simulink library "ammclib_bam"  (Simulink 9.3)
settings: Solver=VariableStepAuto  StartTime=0.0  StopTime=10.0  RelTol=1e-3
undefined symbols (not defined in the file or in its folder): f16A1, f16A2, f16ADCMaxError, f16B0, f16B1, f16B2, f16C1, f16CC1, f16CC1sc, f16CC1sc_D, f16CC1sc_Q, f16CC2, f16CC2sc, f16CC2sc_D, f16CC2sc_Q, f16DerivGain, f16EGain, f16FiltCoef, f16HystOff, f16HystOn, f16IGain, f16IntegGain, f16IntegGainFW, f16IntegGainQ, f16Kd, f16Kq, f16Limit, f16LowerLimit, f16LowerLimit_D, f16LowerLimit_Q, f16LowerLimitFW, f16LowerLimitQ, f16ModIndex, f16OutValOff, f16OutValOn, f16PropGain, f16PropGainFW, f16PropGainQ, f16RampDown, f16RampUp, f16UGain, f16UpperLimit, f16UpperLimit_D, f16UpperLimit_Q, f16UpperLimitFW, f16UpperLimitQ, f16WIGain, f32A1, f32A2, f32ADCMaxError, f32B0, f32B1, f32B2, f32C1, f32CC1, f32CC1sc, f32CC1sc_D, f32CC1sc_Q, f32CC2, f32CC2sc ... (+114)
(part 18 of 21)

== system ammclib_bam/GFLIB/F32/GFLIB_Asin_F32 ==
  f32In : Inport  OutDataTypeStr=int32
  GFLIB_Asin_SF : S-Function  FunctionName=GFLIB_Asin_SF_F32  SFunctionDeploymentMode=off  EnableBusSupport=off
  copyright : Subsystem
      mask Display: text(10,90,'FILE:');text(10,75,'DESRIPTION:');text(10,60,'COPYRIGHT:');text(10,45,'VERSION:');text(10,30,'DATE:')
  copyright2 : Subsystem
      mask Display: text(10,90,'GFLIB_Asin_BAM_F32.mdl');text(10,75,'Inverse sine function');text(10,60,'NXP 2020');text(10,45,'1.0');text(10,30,'18-Mar-2020');
  f32Out : Outport
  wires:
  GFLIB_Asin_SF/1 -> f32Out/1
  f32In/1 -> GFLIB_Asin_SF/1

== system ammclib_bam/GFLIB/F32/GFLIB_AtanYXShifted_F32 ==
  f32InY : Inport  OutDataTypeStr=int32
  f32InX : Inport  Port=2  OutDataTypeStr=int32
  Ky : Inport  Port=3  OutDataTypeStr=int32
  Kx : Inport  Port=4  OutDataTypeStr=int32
  Ny : Inport  Port=5  OutDataTypeStr=int32
  Nx : Inport  Port=6  OutDataTypeStr=int32
  ThetaAdj : Inport  Port=7  OutDataTypeStr=int32
  GFLIB_AtanYXShifted_SF : S-Function  FunctionName=GFLIB_AtanYXShifted_SF_F32  SFunctionDeploymentMode=off  EnableBusSupport=off
  copyright : Subsystem
      mask Display: text(10,90,'FILE:');text(10,75,'DESRIPTION:');text(10,60,'COPYRIGHT:');text(10,45,'VERSION:');text(10,30,'DATE:')
  copyright2 : Subsystem
      mask Display: text(10,90,'GFLIB_AtanYXShifted_BAM_F32.mdl');text(10,75,'Shifted arctangent of two arguments Y/X.');text(10,60,'NXP 2020');text(10,45,'1.0');text(10,30,'18-Mar-2020');
  f32Out : Outport
  wires:
  GFLIB_AtanYXShifted_SF/1 -> f32Out/1
  ThetaAdj/1 -> GFLIB_AtanYXShifted_SF/7
  Nx/1 -> GFLIB_AtanYXShifted_SF/6
  Ny/1 -> GFLIB_AtanYXShifted_SF/5
  Kx/1 -> GFLIB_AtanYXShifted_SF/4
  Ky/1 -> GFLIB_AtanYXShifted_SF/3
  f32InX/1 -> GFLIB_AtanYXShifted_SF/2
  f32InY/1 -> GFLIB_AtanYXShifted_SF/1

== system ammclib_bam/GFLIB/F32/GFLIB_AtanYX_F32 ==
  f32InY : Inport  OutDataTypeStr=int32
  f32InX : Inport  Port=2  OutDataTypeStr=int32
  GFLIB_AtanYX_SF : S-Function  FunctionName=GFLIB_AtanYX_SF_F32  SFunctionDeploymentMode=off  EnableBusSupport=off
  copyright : Subsystem
      mask Display: text(10,90,'FILE:');text(10,75,'DESRIPTION:');text(10,60,'COPYRIGHT:');text(10,45,'VERSION:');text(10,30,'DATE:')
  copyright2 : Subsystem
      mask Display: text(10,90,'GFLIB_AtanYX_BAM_F32.mdl');text(10,75,'Arctangent of two arguments Y/X.');text(10,60,'NXP 2020');text(10,45,'1.0');text(10,30,'18-Mar-2020');
  f32Out : Outport
  wires:
  GFLIB_AtanYX_SF/1 -> f32Out/1
  f32InX/1 -> GFLIB_AtanYX_SF/2
  f32InY/1 -> GFLIB_AtanYX_SF/1

== system ammclib_bam/GFLIB/F32/GFLIB_Atan_F32 ==
  f32In : Inport  OutDataTypeStr=int32
  GFLIB_Atan_SF : S-Function  FunctionName=GFLIB_Atan_SF_F32  SFunctionDeploymentMode=off  EnableBusSupport=off
  copyright : Subsystem
      mask Display: text(10,90,'FILE:');text(10,75,'DESRIPTION:');text(10,60,'COPYRIGHT:');text(10,45,'VERSION:');text(10,30,'DATE:')
  copyright2 : Subsystem
      mask Display: text(10,90,'GFLIB_Atan_BAM_F32.mdl');text(10,75,'Inverse tangent function');text(10,60,'NXP 2020');text(10,45,'1.0');text(10,30,'18-Mar-2020');
  f32Out : Outport
  wires:
  GFLIB_Atan_SF/1 -> f32Out/1
  f32In/1 -> GFLIB_Atan_SF/1

== system ammclib_bam/GFLIB/F32/GFLIB_ControllerPIDpAW_F32 ==
  f32InErr : Inport  OutDataTypeStr=int32
  f32ControllerPIDpAWOut_preset : Inport  Port=2  OutDataTypeStr=int32
  Reset : ResetPort  DisableCoverage=on
  GFLIB_ControllerPIDpAW_SF : S-Function  FunctionName=GFLIB_ControllerPIDpAW_SF_F32  Parameters=showStates,resetStatesEnable,f32PropGain,f32IntegGain,f32DerivGain,f32FiltCoef,s16PropGainShift,s16IntegGainShift,s16DerivGainShift,f32LowerLimit,f32UpperLimit  SFunctionDeploymentMode=off  EnableBusSupport=off
  copyright : Subsystem
      mask Display: text(10,90,'FILE:');text(10,75,'DESRIPTION:');text(10,60,'COPYRIGHT:');text(10,45,'VERSION:');text(10,30,'DATE:')
  copyright2 : Subsystem
      mask Display: text(10,90,'GFLIB_ControllerPIDpAW_BAM_F32.mdl');text(10,75,'Parallel form of a standard PID controller with anti-windup.');text(10,60,'NXP 2020');text(10,45,'1.0');text(10,30,'28-Mar-2020');
  f32DerivGain : Ground
  f32DerivPartK_1 : Ground
  f32DerivPartK_1_Out : Terminator
  f32FiltCoef : Ground
  f32InK_1 : Ground
  f32InK_1_Out : Terminator
  f32IntegGain : Ground
  f32IntegPartK_1 : Ground
  f32IntegPartK_1_Out : Terminator
  f32LowerLimit : Ground
  f32PropGain : Ground
  f32UpperLimit : Ground
  s16DerivGainShift : Ground
  s16IntegGainShift : Ground
  s16PropGainShift : Ground
  f32Out : Outport
  u16LimitFlag : Outport  Port=2
  wires:
  GFLIB_ControllerPIDpAW_SF/5 -> f32InK_1_Out/1
  GFLIB_ControllerPIDpAW_SF/4 -> f32DerivPartK_1_Out/1
  GFLIB_ControllerPIDpAW_SF/3 -> f32IntegPartK_1_Out/1
  GFLIB_ControllerPIDpAW_SF/2 -> u16LimitFlag/1
  GFLIB_ControllerPIDpAW_SF/1 -> f32Out/1
  f32InK_1/1 -> GFLIB_ControllerPIDpAW_SF/14
  f32DerivPartK_1/1 -> GFLIB_ControllerPIDpAW_SF/13
  f32IntegPartK_1/1 -> GFLIB_ControllerPIDpAW_SF/12
  f32UpperLimit/1 -> GFLIB_ControllerPIDpAW_SF/11
  f32LowerLimit/1 -> GFLIB_ControllerPIDpAW_SF/10
  s16DerivGainShift/1 -> GFLIB_ControllerPIDpAW_SF/9
  s16IntegGainShift/1 -> GFLIB_ControllerPIDpAW_SF/8
  s16PropGainShift/1 -> GFLIB_ControllerPIDpAW_SF/7
  f32FiltCoef/1 -> GFLIB_ControllerPIDpAW_SF/6
  f32DerivGain/1 -> GFLIB_ControllerPIDpAW_SF/5
  f32IntegGain/1 -> GFLIB_ControllerPIDpAW_SF/4
  f32PropGain/1 -> GFLIB_ControllerPIDpAW_SF/3
  f32ControllerPIDpAWOut_preset/1 -> GFLIB_ControllerPIDpAW_SF/2
  f32InErr/1 -> GFLIB_ControllerPIDpAW_SF/1

== system ammclib_bam/GFLIB/F32/GFLIB_ControllerPIpAW_F32 ==
  f32InErr : Inport  OutDataTypeStr=int32
  f32ControllerPIpAWOut_preset : Inport  Port=2  OutDataTypeStr=int32
  Reset : ResetPort  DisableCoverage=on
  GFLIB_ControllerPIpAW_SF : S-Function  FunctionName=GFLIB_ControllerPIpAW_SF_F32  Parameters=showStates,resetStatesEnable,f32PropGain,f32IntegGain,s16PropGainShift,s16IntegGainShift,f32LowerLimit,f32UpperLimit  SFunctionDeploymentMode=off  EnableBusSupport=off
  copyright : Subsystem
      mask Display: text(10,90,'FILE:');text(10,75,'DESRIPTION:');text(10,60,'COPYRIGHT:');text(10,45,'VERSION:');text(10,30,'DATE:')
  copyright2 : Subsystem
      mask Display: text(10,90,'GFLIB_ControllerPIpAW_BAM_F32.mdl');text(10,75,'Parallel form of a standard PI controller with anti-windup.');text(10,60,'NXP 2020');text(10,45,'1.0');text(10,30,'28-Mar-2020');
  f32InK_1 : Ground
  f32InK_1_Out : Terminator
  f32IntegGain : Ground
  f32IntegPartK_1 : Ground
  f32IntegPartK_1_Out : Terminator
  f32LowerLimit : Ground
  f32PropGain : Ground
  f32UpperLimit : Ground
  s16IntegGainShift : Ground
  s16PropGainShift : Ground
  f32Out : Outport
  u16LimitFlag : Outport  Port=2
  wires:
  GFLIB_ControllerPIpAW_SF/4 -> f32InK_1_Out/1
  GFLIB_ControllerPIpAW_SF/3 -> f32IntegPartK_1_Out/1
  GFLIB_ControllerPIpAW_SF/2 -> u16LimitFlag/1
  GFLIB_ControllerPIpAW_SF/1 -> f32Out/1
  f32InK_1/1 -> GFLIB_ControllerPIpAW_SF/10
  f32IntegPartK_1/1 -> GFLIB_ControllerPIpAW_SF/9
  f32UpperLimit/1 -> GFLIB_ControllerPIpAW_SF/8
  f32LowerLimit/1 -> GFLIB_ControllerPIpAW_SF/7
  s16IntegGainShift/1 -> GFLIB_ControllerPIpAW_SF/6
  s16PropGainShift/1 -> GFLIB_ControllerPIpAW_SF/5
  f32IntegGain/1 -> GFLIB_ControllerPIpAW_SF/4
  f32PropGain/1 -> GFLIB_ControllerPIpAW_SF/3
  f32ControllerPIpAWOut_preset/1 -> GFLIB_ControllerPIpAW_SF/2
  f32InErr/1 -> GFLIB_ControllerPIpAW_SF/1

== system ammclib_bam/GFLIB/F32/GFLIB_ControllerPIp_F32 ==
  f32InErr : Inport  OutDataTypeStr=int32
  f32ControllerPIpOut_preset : Inport  Port=2  OutDataTypeStr=int32
  Reset : ResetPort  DisableCoverage=on
  GFLIB_ControllerPIp_SF : S-Function  FunctionName=GFLIB_ControllerPIp_SF_F32  Parameters=showStates,resetStatesEnable,f32PropGain,f32IntegGain,s16PropGainShift,s16IntegGainShift  SFunctionDeploymentMode=off  EnableBusSupport=off
  copyright : Subsystem
      mask Display: text(10,90,'FILE:');text(10,75,'DESRIPTION:');text(10,60,'COPYRIGHT:');text(10,45,'VERSION:');text(10,30,'DATE:')
  copyright2 : Subsystem
      mask Display: text(10,90,'GFLIB_ControllerPIp_BAM_F32.mdl');text(10,75,'Parallel form of a standard PI controller without anti-windup.');text(10,60,'NXP 2020');text(10,45,'1.0');text(10,30,'28-Mar-2020');
  f32InK_1 : Ground
  f32InK_1_Out : Terminator
  f32IntegGain : Ground
  f32IntegPartK_1 : Ground
  f32IntegPartK_1_Out : Terminator
  f32PropGain : Ground
  s16IntegGainShift : Ground
  s16PropGainShift : Ground
  f32Out : Outport
  wires:
  GFLIB_ControllerPIp_SF/3 -> f32InK_1_Out/1
  GFLIB_ControllerPIp_SF/2 -> f32IntegPartK_1_Out/1
  GFLIB_ControllerPIp_SF/1 -> f32Out/1
  f32InK_1/1 -> GFLIB_ControllerPIp_SF/8
  f32IntegPartK_1/1 -> GFLIB_ControllerPIp_SF/7
  s16IntegGainShift/1 -> GFLIB_ControllerPIp_SF/6
  s16PropGainShift/1 -> GFLIB_ControllerPIp_SF/5
  f32IntegGain/1 -> GFLIB_ControllerPIp_SF/4
  f32PropGain/1 -> GFLIB_ControllerPIp_SF/3
  f32ControllerPIpOut_preset/1 -> GFLIB_ControllerPIp_SF/2
  f32InErr/1 -> GFLIB_ControllerPIp_SF/1

== system ammclib_bam/GFLIB/F32/GFLIB_ControllerPIrAW_F32 ==
  f32InErr : Inport  OutDataTypeStr=int32
  f32ControllerPIrAWOut_preset : Inport  Port=2  OutDataTypeStr=int32
  Reset : ResetPort  DisableCoverage=on
  GFLIB_ControllerPIrAW_SF : S-Function  FunctionName=GFLIB_ControllerPIrAW_SF_F32  Parameters=showStates,resetStatesEnable,f32UpperLimit,f32LowerLimit,f32CC1sc,f32CC2sc,u16NShift  SFunctionDeploymentMode=off  EnableBusSupport=off
  copyright : Subsystem
      mask Display: text(10,90,'FILE:');text(10,75,'DESRIPTION:');text(10,60,'COPYRIGHT:');text(10,45,'VERSION:');text(10,30,'DATE:')
  copyright2 : Subsystem
      mask Display: text(10,90,'GFLIB_ControllerPIrAW_BAM_F32.mdl');text(10,75,'Recurrent form PI controller with anti-windup.');text(10,60,'NXP 2020');text(10,45,'1.0');text(10,30,'28-Mar-2020');
  f32Acc : Ground
  f32Acc_Out : Terminator
  f32CC1sc : Ground
  f32CC2sc : Ground
  f32InErrK1 : Ground
  f32InErrK1_Out : Terminator
  f32LowerLimit : Ground
  f32UpperLimit : Ground
  u16NShift : Ground
  f32Out : Outport
  wires:
  GFLIB_ControllerPIrAW_SF/3 -> f32InErrK1_Out/1
  GFLIB_ControllerPIrAW_SF/2 -> f32Acc_Out/1
  GFLIB_ControllerPIrAW_SF/1 -> f32Out/1
  u16NShift/1 -> GFLIB_ControllerPIrAW_SF/9
  f32CC2sc/1 -> GFLIB_ControllerPIrAW_SF/8
  f32CC1sc/1 -> GFLIB_ControllerPIrAW_SF/7
  f32InErrK1/1 -> GFLIB_ControllerPIrAW_SF/6
  f32Acc/1 -> GFLIB_ControllerPIrAW_SF/5
  f32LowerLimit/1 -> GFLIB_ControllerPIrAW_SF/4
  f32UpperLimit/1 -> GFLIB_ControllerPIrAW_SF/3
  f32ControllerPIrAWOut_preset/1 -> GFLIB_ControllerPIrAW_SF/2
  f32InErr/1 -> GFLIB_ControllerPIrAW_SF/1

== system ammclib_bam/GFLIB/F32/GFLIB_ControllerPIr_F32 ==
  f32InErr : Inport  OutDataTypeStr=int32
  f32ControllerPIrOut_preset : Inport  Port=2  OutDataTypeStr=int32
  Reset : ResetPort  DisableCoverage=on
  GFLIB_ControllerPIr_SF : S-Function  FunctionName=GFLIB_ControllerPIr_SF_F32  Parameters=showStates,resetStatesEnable,f32CC1,f32CC2,u16NShift  SFunctionDeploymentMode=off  EnableBusSupport=off
  copyright : Subsystem
      mask Display: text(10,90,'FILE:');text(10,75,'DESRIPTION:');text(10,60,'COPYRIGHT:');text(10,45,'VERSION:');text(10,30,'DATE:')
  copyright2 : Subsystem
      mask Display: text(10,90,'GFLIB_ControllerPIr_BAM_F32.mdl');text(10,75,'Recurrent form PI controller without anti-windup.');text(10,60,'NXP 2020');text(10,45,'1.0');text(10,30,'28-Mar-2020');
  f32Acc : Ground
  f32Acc_Out : Terminator
  f32CC1sc : Ground
  f32CC2sc : Ground
  f32InErrK1 : Ground
  f32InErrK1_Out : Terminator
  u16NShift : Ground
  f32Out : Outport
  wires:
  GFLIB_ControllerPIr_SF/3 -> f32InErrK1_Out/1
  GFLIB_ControllerPIr_SF/2 -> f32Acc_Out/1
  GFLIB_ControllerPIr_SF/1 -> f32Out/1
  u16NShift/1 -> GFLIB_ControllerPIr_SF/7
  f32InErrK1/1 -> GFLIB_ControllerPIr_SF/6
  f32Acc/1 -> GFLIB_ControllerPIr_SF/5
  f32CC2sc/1 -> GFLIB_ControllerPIr_SF/4
  f32CC1sc/1 -> GFLIB_ControllerPIr_SF/3
  f32ControllerPIrOut_preset/1 -> GFLIB_ControllerPIr_SF/2
  f32InErr/1 -> GFLIB_ControllerPIr_SF/1

== system ammclib_bam/GFLIB/F32/GFLIB_Cos_F32 ==
  f32In : Inport  OutDataTypeStr=int32
  GFLIB_Cos_SF : S-Function  FunctionName=GFLIB_Cos_SF_F32  SFunctionDeploymentMode=off  EnableBusSupport=off
  copyright : Subsystem
      mask Display: text(10,90,'FILE:');text(10,75,'DESRIPTION:');text(10,60,'COPYRIGHT:');text(10,45,'VERSION:');text(10,30,'DATE:')
  copyright2 : Subsystem
      mask Display: text(10,90,'GFLIB_Cos_BAM_F32.mdl');text(10,75,'Cosine function');text(10,60,'NXP 2020');text(10,45,'1.0');text(10,30,'18-Mar-2020');
  f32Out : Outport
  wires:
  GFLIB_Cos_SF/1 -> f32Out/1
  f32In/1 -> GFLIB_Cos_SF/1

== system ammclib_bam/GFLIB/F32/GFLIB_Hyst_F32 ==
  f32In : Inport  OutDataTypeStr=int32
  GFLIB_Hyst_SF : S-Function  FunctionName=GFLIB_Hyst_SF_F32  Parameters=showStates,f32HystOn,f32HystOff,f32OutValOn,f32OutValOff  SFunctionDeploymentMode=off  EnableBusSupport=off
  copyright : Subsystem
      mask Display: text(10,90,'FILE:');text(10,75,'DESRIPTION:');text(10,60,'COPYRIGHT:');text(10,45,'VERSION:');text(10,30,'DATE:')
  copyright2 : Subsystem
      mask Display: text(10,90,'GFLIB_Hyst_BAM_F32.mdl');text(10,75,'Hysteresis function.');text(10,60,'NXP 2020');text(10,45,'1.0');text(10,30,'18-Mar-2020');
  f32HystOff : Ground
  f32HystOn : Ground
  f32OutState : Ground
  f32OutState_Out : Terminator
  f32OutValOff : Ground
  f32OutValOn : Ground
  f32Out : Outport
  wires:
  GFLIB_Hyst_SF/2 -> f32OutState_Out/1
  GFLIB_Hyst_SF/1 -> f32Out/1
  f32OutState/1 -> GFLIB_Hyst_SF/6
  f32OutValOff/1 -> GFLIB_Hyst_SF/5
  f32OutValOn/1 -> GFLIB_Hyst_SF/4
  f32HystOff/1 -> GFLIB_Hyst_SF/3
  f32HystOn/1 -> GFLIB_Hyst_SF/2
  f32In/1 -> GFLIB_Hyst_SF/1

== system ammclib_bam/GFLIB/F32/GFLIB_IntegratorTR_F32 ==
  f32In : Inport  OutDataTypeStr=int32
  f32IntegratorTROut_preset : Inport  Port=2  OutDataTypeStr=int32
  Reset : ResetPort  DisableCoverage=on
  GFLIB_IntegratorTR_SF : S-Function  FunctionName=GFLIB_IntegratorTR_SF_F32  Parameters=showStates,resetStatesEnable,f32C1,u16NShift  SFunctionDeploymentMode=off  EnableBusSupport=off
  copyright : Subsystem
      mask Display: text(10,90,'FILE:');text(10,75,'DESRIPTION:');text(10,60,'COPYRIGHT:');text(10,45,'VERSION:');text(10,30,'DATE:')
  copyright2 : Subsystem
      mask Display: text(10,90,'GFLIB_IntegratorTR_BAM_F32.mdl');text(10,75,'Discrete integrator transformed from a linear model using Billinear (trapezoidal) transformation.');text(10,60,'NXP 2020');text(10,45,'1.0');text(10,30,'28-Mar-2020');
  f32C1 : Ground
  f32InK1 : Ground
  f32InK1_Out : Terminator
  f32State : Ground
  f32State_Out : Terminator
  u16NShift : Ground
  f32Out : Outport
  wires:
  GFLIB_IntegratorTR_SF/3 -> f32InK1_Out/1
  GFLIB_IntegratorTR_SF/2 -> f32State_Out/1
  GFLIB_IntegratorTR_SF/1 -> f32Out/1
  f32InK1/1 -> GFLIB_IntegratorTR_SF/6
  f32State/1 -> GFLIB_IntegratorTR_SF/5
  u16NShift/1 -> GFLIB_IntegratorTR_SF/4
  f32C1/1 -> GFLIB_IntegratorTR_SF/3
  f32IntegratorTROut_preset/1 -> GFLIB_IntegratorTR_SF/2
  f32In/1 -> GFLIB_IntegratorTR_SF/1

== system ammclib_bam/GFLIB/F32/GFLIB_Limit_F32 ==
  f32In : Inport  OutDataTypeStr=int32
  GFLIB_Limit_SF : S-Function  FunctionName=GFLIB_Limit_SF_F32  Parameters=showStates,f32LowerLimit,f32UpperLimit  SFunctionDeploymentMode=off  EnableBusSupport=off
  copyright : Subsystem
      mask Display: text(10,90,'FILE:');text(10,75,'DESRIPTION:');text(10,60,'COPYRIGHT:');text(10,45,'VERSION:');text(10,30,'DATE:')
  copyright2 : Subsystem
      mask Display: text(10,90,'GFLIB_Limit_BAM_F32.mdl');text(10,75,'Limit function.');text(10,60,'NXP 2020');text(10,45,'1.0');text(10,30,'23-Mar-2020');
  f32LowerLimit : Ground
  f32UpperLimit : Ground
  f32Out : Outport
  wires:
  GFLIB_Limit_SF/1 -> f32Out/1
  f32UpperLimit/1 -> GFLIB_Limit_SF/3
  f32LowerLimit/1 -> GFLIB_Limit_SF/2
  f32In/1 -> GFLIB_Limit_SF/1

== system ammclib_bam/GFLIB/F32/GFLIB_LowerLimit_F32 ==
  f32In : Inport  OutDataTypeStr=int32
  GFLIB_LowerLimit_SF : S-Function  FunctionName=GFLIB_LowerLimit_SF_F32  Parameters=showStates,f32LowerLimit  SFunctionDeploymentMode=off  EnableBusSupport=off
  copyright : Subsystem
      mask Display: text(10,90,'FILE:');text(10,75,'DESRIPTION:');text(10,60,'COPYRIGHT:');text(10,45,'VERSION:');text(10,30,'DATE:')
  copyright2 : Subsystem
      mask Display: text(10,90,'GFLIB_LowerLimit_BAM_F32.mdl');text(10,75,'Lower limit function.');text(10,60,'NXP 2020');text(10,45,'1.0');text(10,30,'18-Mar-2020');
  f32LowerLimit : Ground
  f32Out : Outport
  wires:
  GFLIB_LowerLimit_SF/1 -> f32Out/1
  f32LowerLimit/1 -> GFLIB_LowerLimit_SF/2
  f32In/1 -> GFLIB_LowerLimit_SF/1

== system ammclib_bam/GFLIB/F32/GFLIB_Lut1D_F32 ==
  f32In : Inport  OutDataTypeStr=int32
  u32ShamOffset : Inport  Port=2  OutDataTypeStr=uint32
  GFLIB_Lut1D_SF : S-Function  FunctionName=GFLIB_Lut1D_SF_F32  Parameters=pf32Table,s32MidIdx  SFunctionDeploymentMode=off  EnableBusSupport=off
  copyright : Subsystem
      mask Display: text(10,90,'FILE:');text(10,75,'DESRIPTION:');text(10,60,'COPYRIGHT:');text(10,45,'VERSION:');text(10,30,'DATE:')
  copyright2 : Subsystem
      mask Display: text(10,90,'GFLIB_Lut1D_BAM_F32.mdl');text(10,75,'One dimensional lookup table function');text(10,60,'NXP 2020');text(10,45,'1.0');text(10,30,'23-Mar-2020');
  f32Out : Outport
  wires:
  GFLIB_Lut1D_SF/1 -> f32Out/1
  u32ShamOffset/1 -> GFLIB_Lut1D_SF/2
  f32In/1 -> GFLIB_Lut1D_SF/1

== system ammclib_bam/GFLIB/F32/GFLIB_Lut2D_F32 ==
  f32In1 : Inport  OutDataTypeStr=int32
  f32In2 : Inport  Port=2  OutDataTypeStr=int32
  u32ShamOffset1 : Inport  Port=3  OutDataTypeStr=uint32
  u32ShamOffset2 : Inport  Port=4  OutDataTypeStr=uint32
  GFLIB_Lut2D_SF : S-Function  FunctionName=GFLIB_Lut2D_SF_F32  Parameters=pf32Table,s32MidIdx  SFunctionDeploymentMode=off  EnableBusSupport=off
  copyright : Subsystem
      mask Display: text(10,90,'FILE:');text(10,75,'DESRIPTION:');text(10,60,'COPYRIGHT:');text(10,45,'VERSION:');text(10,30,'DATE:')
  copyright2 : Subsystem
      mask Display: text(10,90,'GFLIB_Lut2D_BAM_F32.mdl');text(10,75,'Two dimensional lookup table function');text(10,60,'NXP 2020');text(10,45,'1.0');text(10,30,'23-Mar-2020');
  f32Out : Outport
  wires:
  GFLIB_Lut2D_SF/1 -> f32Out/1
  u32ShamOffset2/1 -> GFLIB_Lut2D_SF/4
  u32ShamOffset1/1 -> GFLIB_Lut2D_SF/3
  f32In2/1 -> GFLIB_Lut2D_SF/2
  f32In1/1 -> GFLIB_Lut2D_SF/1

== system ammclib_bam/GFLIB/F32/GFLIB_Ramp_F32 ==
  f32In : Inport  OutDataTypeStr=int32
  GFLIB_Ramp_SF : S-Function  FunctionName=GFLIB_Ramp_SF_F32  Parameters=showStates,f32RampUp,f32RampDown  SFunctionDeploymentMode=off  EnableBusSupport=off
  copyright : Subsystem
      mask Display: text(10,90,'FILE:');text(10,75,'DESRIPTION:');text(10,60,'COPYRIGHT:');text(10,45,'VERSION:');text(10,30,'DATE:')
  copyright2 : Subsystem
      mask Display: text(10,90,'GFLIB_Ramp_BAM_F32.mdl');text(10,75,'Rate of change limiter - ramp function.');text(10,60,'NXP 2020');text(10,45,'1.0');text(10,30,'18-Mar-2020');
  f32RampDown : Ground
  f32RampUp : Ground
  f32State : Ground
  f32State_Out : Terminator
  f32Out : Outport
  wires:
  GFLIB_Ramp_SF/2 -> f32State_Out/1
  GFLIB_Ramp_SF/1 -> f32Out/1
  f32RampDown/1 -> GFLIB_Ramp_SF/4
  f32RampUp/1 -> GFLIB_Ramp_SF/3
  f32State/1 -> GFLIB_Ramp_SF/2
  f32In/1 -> GFLIB_Ramp_SF/1

== system ammclib_bam/GFLIB/F32/GFLIB_Sign_F32 ==
  f32In : Inport  OutDataTypeStr=int32
  GFLIB_Sign_SF : S-Function  FunctionName=GFLIB_Sign_SF_F32  SFunctionDeploymentMode=off  EnableBusSupport=off
  copyright : Subsystem
      mask Display: text(10,90,'FILE:');text(10,75,'DESRIPTION:');text(10,60,'COPYRIGHT:');text(10,45,'VERSION:');text(10,30,'DATE:')
  copyright2 : Subsystem
      mask Display: text(10,90,'GFLIB_Sign_BAM_F32.mdl');text(10,75,'Sign function.');text(10,60,'NXP 2020');text(10,45,'1.0');text(10,30,'18-Mar-2020');
  f32Out : Outport
  wires:
  GFLIB_Sign_SF/1 -> f32Out/1
  f32In/1 -> GFLIB_Sign_SF/1

== system ammclib_bam/GFLIB/F32/GFLIB_SinCos_F32 ==
  f32In : Inport  OutDataTypeStr=int32
  GFLIB_SinCos_SF : S-Function  FunctionName=GFLIB_SinCos_SF_F32  SFunctionDeploymentMode=off  EnableBusSupport=off
  copyright : Subsystem
      mask Display: text(10,90,'FILE:');text(10,75,'DESRIPTION:');text(10,60,'COPYRIGHT:');text(10,45,'VERSION:');text(10,30,'DATE:')
  copyright2 : Subsystem
      mask Display: text(10,90,'GFLIB_SinCos_BAM_F32.mdl');text(10,75,'Sine and cosine of the same argument');text(10,60,'NXP 2020');text(10,45,'1.0');text(10,30,'18-Mar-2020');
  pOut : Outport
  wires:
  GFLIB_SinCos_SF/1 -> pOut/1
  f32In/1 -> GFLIB_SinCos_SF/1

== system ammclib_bam/GFLIB/F32/GFLIB_Sin_F32 ==
  f32In : Inport  OutDataTypeStr=int32
  GFLIB_Sin_SF : S-Function  FunctionName=GFLIB_Sin_SF_F32  SFunctionDeploymentMode=off  EnableBusSupport=off
  copyright : Subsystem
      mask Display: text(10,90,'FILE:');text(10,75,'DESRIPTION:');text(10,60,'COPYRIGHT:');text(10,45,'VERSION:');text(10,30,'DATE:')
  copyright2 : Subsystem
      mask Display: text(10,90,'GFLIB_Sin_BAM_F32.mdl');text(10,75,'Sine function');text(10,60,'NXP 2020');text(10,45,'1.0');text(10,30,'18-Mar-2020');
  f32Out : Outport
  wires:
  GFLIB_Sin_SF/1 -> f32Out/1
  f32In/1 -> GFLIB_Sin_SF/1

== system ammclib_bam/GFLIB/F32/GFLIB_Sqrt_F32 ==
  f32In : Inport  OutDataTypeStr=int32
  GFLIB_Sqrt_SF : S-Function  FunctionName=GFLIB_Sqrt_SF_F32  SFunctionDeploymentMode=off  EnableBusSupport=off
  copyright : Subsystem
      mask Display: text(10,90,'FILE:');text(10,75,'DESRIPTION:');text(10,60,'COPYRIGHT:');text(10,45,'VERSION:');text(10,30,'DATE:')
  copyright2 : Subsystem
      mask Display: text(10,90,'GFLIB_Sqrt_BAM_F32.mdl');text(10,75,'Square root approximation.');text(10,60,'NXP 2020');text(10,45,'1.0');text(10,30,'18-Mar-2020');
  f32Out : Outport
  wires:
  GFLIB_Sqrt_SF/1 -> f32Out/1
  f32In/1 -> GFLIB_Sqrt_SF/1

== system ammclib_bam/GFLIB/F32/GFLIB_Tan_F32 ==
  f32In : Inport  OutDataTypeStr=int32
  GFLIB_Tan_SF : S-Function  FunctionName=GFLIB_Tan_SF_F32  SFunctionDeploymentMode=off  EnableBusSupport=off
  copyright : Subsystem
      mask Display: text(10,90,'FILE:');text(10,75,'DESRIPTION:');text(10,60,'COPYRIGHT:');text(10,45,'VERSION:');text(10,30,'DATE:')
  copyright2 : Subsystem
      mask Display: text(10,90,'GFLIB_Tan_BAM_F32.mdl');text(10,75,'Trigonometric tangent function');text(10,60,'NXP 2020');text(10,45,'1.0');text(10,30,'18-Mar-2020');
  f32Out : Outport
  wires:
  GFLIB_Tan_SF/1 -> f32Out/1
  f32In/1 -> GFLIB_Tan_SF/1

== system ammclib_bam/GFLIB/F32/GFLIB_UpperLimit_F32 ==
  f32In : Inport  OutDataTypeStr=int32
  GFLIB_UpperLimit_SF : S-Function  FunctionName=GFLIB_UpperLimit_SF_F32  Parameters=showStates,f32UpperLimit  SFunctionDeploymentMode=off  EnableBusSupport=off
  copyright : Subsystem
      mask Display: text(10,90,'FILE:');text(10,75,'DESRIPTION:');text(10,60,'COPYRIGHT:');text(10,45,'VERSION:');text(10,30,'DATE:')
  copyright2 : Subsystem
      mask Display: text(10,90,'GFLIB_UpperLimit_BAM_F32.mdl');text(10,75,'Upper limit function.');text(10,60,'NXP 2020');text(10,45,'1.0');text(10,30,'23-Mar-2020');
  f32UpperLimit : Ground
  f32Out : Outport
  wires:
  GFLIB_UpperLimit_SF/1 -> f32Out/1
  f32UpperLimit/1 -> GFLIB_UpperLimit_SF/2
  f32In/1 -> GFLIB_UpperLimit_SF/1

== system ammclib_bam/GFLIB/F32/GFLIB_VMin_F32 ==
  pIn : Inport  OutDataTypeStr=int32
  GFLIB_VMin_SF : S-Function  FunctionName=GFLIB_VMin_SF_F32  SFunctionDeploymentMode=off  EnableBusSupport=off
  copyright : Subsystem
      mask Display: text(10,90,'FILE:');text(10,75,'DESRIPTION:');text(10,60,'COPYRIGHT:');text(10,45,'VERSION:');text(10,30,'DATE:')
  copyright2 : Subsystem
      mask Display: text(10,90,'GFLIB_VMin_BAM_F32.mdl');text(10,75,'Vector minimum');text(10,60,'NXP 2020');text(10,45,'1.0');text(10,30,'18-Mar-2020');
  IndexOfMinimum : Outport
  wires:
  GFLIB_VMin_SF/1 -> IndexOfMinimum/1
  pIn/1 -> GFLIB_VMin_SF/1

== system ammclib_bam/GFLIB/F32/GFLIB_VectorLimit_F32 ==
  pIn : Inport  OutDataTypeStr=Bus: SWLIBS_2Syst_F32  BusOutputAsStruct=on
  GFLIB_VectorLimit_SF : S-Function  FunctionName=GFLIB_VectorLimit_SF_F32  Parameters=showStates,f32Limit  SFunctionDeploymentMode=off  EnableBusSupport=off
  copyright : Subsystem
      mask Display: text(10,90,'FILE:');text(10,75,'DESRIPTION:');text(10,60,'COPYRIGHT:');text(10,45,'VERSION:');text(10,30,'DATE:')
  copyright2 : Subsystem
      mask Display: text(10,90,'GFLIB_VectorLimit_BAM_F32.mdl');text(10,75,'Vector Limit function.');text(10,60,'NXP 2020');text(10,45,'1.0');text(10,30,'18-Mar-2020');
  f32Limit : Ground
  bFlag : Outport
  pOut : Outport  Port=2
  wires:
  GFLIB_VectorLimit_SF/2 -> pOut/1
  GFLIB_VectorLimit_SF/1 -> bFlag/1
  f32Limit/1 -> GFLIB_VectorLimit_SF/2
  pIn/1 -> GFLIB_VectorLimit_SF/1

== system ammclib_bam/GFLIB/FLT/GFLIB_Acos_FLT ==
  fltIn : Inport  OutDataTypeStr=single
  GFLIB_Acos_SF : S-Function  FunctionName=GFLIB_Acos_SF_FLT  SFunctionDeploymentMode=off  EnableBusSupport=off
  copyright : Subsystem
      mask Display: text(10,90,'FILE:');text(10,75,'DESRIPTION:');text(10,60,'COPYRIGHT:');text(10,45,'VERSION:');text(10,30,'DATE:')
  copyright2 : Subsystem
      mask Display: text(10,90,'GFLIB_Acos_BAM_FLT.mdl');text(10,75,'Inverse cosine function');text(10,60,'NXP 2020');text(10,45,'1.0');text(10,30,'18-Mar-2020');
  fltOut : Outport
  wires:
  GFLIB_Acos_SF/1 -> fltOut/1
  fltIn/1 -> GFLIB_Acos_SF/1

== system ammclib_bam/GFLIB/FLT/GFLIB_Asin_FLT ==
  fltIn : Inport  OutDataTypeStr=single
  GFLIB_Asin_SF : S-Function  FunctionName=GFLIB_Asin_SF_FLT  SFunctionDeploymentMode=off  EnableBusSupport=off
  copyright : Subsystem
      mask Display: text(10,90,'FILE:');text(10,75,'DESRIPTION:');text(10,60,'COPYRIGHT:');text(10,45,'VERSION:');text(10,30,'DATE:')
  copyright2 : Subsystem
      mask Display: text(10,90,'GFLIB_Asin_BAM_FLT.mdl');text(10,75,'Inverse sine function');text(10,60,'NXP 2020');text(10,45,'1.0');text(10,30,'18-Mar-2020');
  fltOut : Outport
  wires:
  GFLIB_Asin_SF/1 -> fltOut/1
  fltIn/1 -> GFLIB_Asin_SF/1

== system ammclib_bam/GFLIB/FLT/GFLIB_AtanYXShifted_FLT ==
  fltInY : Inport  OutDataTypeStr=single
  fltInX : Inport  Port=2  OutDataTypeStr=single
  Ky : Inport  Port=3  OutDataTypeStr=single
  Kx : Inport  Port=4  OutDataTypeStr=single
  ThetaAdj : Inport  Port=5  OutDataTypeStr=single
  GFLIB_AtanYXShifted_SF : S-Function  FunctionName=GFLIB_AtanYXShifted_SF_FLT  SFunctionDeploymentMode=off  EnableBusSupport=off
  copyright : Subsystem
      mask Display: text(10,90,'FILE:');text(10,75,'DESRIPTION:');text(10,60,'COPYRIGHT:');text(10,45,'VERSION:');text(10,30,'DATE:')
  copyright2 : Subsystem
      mask Display: text(10,90,'GFLIB_AtanYXShifted_BAM_FLT.mdl');text(10,75,'Shifted arctangent of two arguments Y/X.');text(10,60,'NXP 2020');text(10,45,'1.0');text(10,30,'18-Mar-2020');
  fltOut : Outport
  wires:
  GFLIB_AtanYXShifted_SF/1 -> fltOut/1
  ThetaAdj/1 -> GFLIB_AtanYXShifted_SF/5
  Kx/1 -> GFLIB_AtanYXShifted_SF/4
  Ky/1 -> GFLIB_AtanYXShifted_SF/3
  fltInX/1 -> GFLIB_AtanYXShifted_SF/2
  fltInY/1 -> GFLIB_AtanYXShifted_SF/1

== system ammclib_bam/GFLIB/FLT/GFLIB_AtanYX_FLT ==
  fltInY : Inport  OutDataTypeStr=single
  fltInX : Inport  Port=2  OutDataTypeStr=single
  GFLIB_AtanYX_SF : S-Function  FunctionName=GFLIB_AtanYX_SF_FLT  SFunctionDeploymentMode=off  EnableBusSupport=off
  copyright : Subsystem
      mask Display: text(10,90,'FILE:');text(10,75,'DESRIPTION:');text(10,60,'COPYRIGHT:');text(10,45,'VERSION:');text(10,30,'DATE:')
  copyright2 : Subsystem
      mask Display: text(10,90,'GFLIB_AtanYX_BAM_FLT.mdl');text(10,75,'Arctangent of two arguments Y/X.');text(10,60,'NXP 2020');text(10,45,'1.0');text(10,30,'18-Mar-2020');
  fltOut : Outport
  wires:
  GFLIB_AtanYX_SF/1 -> fltOut/1
  fltInX/1 -> GFLIB_AtanYX_SF/2
  fltInY/1 -> GFLIB_AtanYX_SF/1

== system ammclib_bam/GFLIB/FLT/GFLIB_Atan_FLT ==
  fltIn : Inport  OutDataTypeStr=single
  GFLIB_Atan_SF : S-Function  FunctionName=GFLIB_Atan_SF_FLT  SFunctionDeploymentMode=off  EnableBusSupport=off
  copyright : Subsystem
      mask Display: text(10,90,'FILE:');text(10,75,'DESRIPTION:');text(10,60,'COPYRIGHT:');text(10,45,'VERSION:');text(10,30,'DATE:')
  copyright2 : Subsystem
      mask Display: text(10,90,'GFLIB_Atan_BAM_FLT.mdl');text(10,75,'Inverse tangent function');text(10,60,'NXP 2020');text(10,45,'1.0');text(10,30,'18-Mar-2020');
  fltOut : Outport
  wires:
  GFLIB_Atan_SF/1 -> fltOut/1
  fltIn/1 -> GFLIB_Atan_SF/1

== system ammclib_bam/GFLIB/FLT/GFLIB_ControllerPIDpAW_FLT ==
  fltInErr : Inport  OutDataTypeStr=single
  fltControllerPIDpAWOut_preset : Inport  Port=2  OutDataTypeStr=single
  Reset : ResetPort  DisableCoverage=on
  GFLIB_ControllerPIDpAW_SF : S-Function  FunctionName=GFLIB_ControllerPIDpAW_SF_FLT  Parameters=showStates,resetStatesEnable,fltPropGain,fltIntegGain,fltDerivGain,fltFiltCoef,fltLowerLimit,fltUpperLimit  SFunctionDeploymentMode=off  EnableBusSupport=off
  copyright : Subsystem
      mask Display: text(10,90,'FILE:');text(10,75,'DESRIPTION:');text(10,60,'COPYRIGHT:');text(10,45,'VERSION:');text(10,30,'DATE:')
  copyright2 : Subsystem
      mask Display: text(10,90,'GFLIB_ControllerPIDpAW_BAM_FLT.mdl');text(10,75,'Parallel form of a standard PID controller with anti-windup.');text(10,60,'NXP 2020');text(10,45,'1.0');text(10,30,'28-Mar-2020');
  fltDerivGain : Ground
  fltDerivPartK_1 : Ground
  fltDerivPartK_1_Out : Terminator
  fltFiltCoef : Ground
  fltInK_1 : Ground
  fltInK_1_Out : Terminator
  fltIntegGain : Ground
  fltIntegPartK_1 : Ground
  fltIntegPartK_1_Out : Terminator
  fltLowerLimit : Ground
  fltPropGain : Ground
  fltUpperLimit : Ground
  fltOut : Outport
  u16LimitFlag : Outport  Port=2
  wires:
  GFLIB_ControllerPIDpAW_SF/5 -> fltInK_1_Out/1
  GFLIB_ControllerPIDpAW_SF/4 -> fltDerivPartK_1_Out/1
  GFLIB_ControllerPIDpAW_SF/3 -> fltIntegPartK_1_Out/1
  GFLIB_ControllerPIDpAW_SF/2 -> u16LimitFlag/1
  GFLIB_ControllerPIDpAW_SF/1 -> fltOut/1
  fltInK_1/1 -> GFLIB_ControllerPIDpAW_SF/11
  fltDerivPartK_1/1 -> GFLIB_ControllerPIDpAW_SF/10
  fltIntegPartK_1/1 -> GFLIB_ControllerPIDpAW_SF/9
  fltUpperLimit/1 -> GFLIB_ControllerPIDpAW_SF/8
  fltLowerLimit/1 -> GFLIB_ControllerPIDpAW_SF/7
  fltFiltCoef/1 -> GFLIB_ControllerPIDpAW_SF/6
  fltDerivGain/1 -> GFLIB_ControllerPIDpAW_SF/5
  fltIntegGain/1 -> GFLIB_ControllerPIDpAW_SF/4
  fltPropGain/1 -> GFLIB_ControllerPIDpAW_SF/3
  fltControllerPIDpAWOut_preset/1 -> GFLIB_ControllerPIDpAW_SF/2
  fltInErr/1 -> GFLIB_ControllerPIDpAW_SF/1

== system ammclib_bam/GFLIB/FLT/GFLIB_ControllerPIpAW_FLT ==
  fltInErr : Inport  OutDataTypeStr=single
  fltControllerPIpAWOut_preset : Inport  Port=2  OutDataTypeStr=single
  Reset : ResetPort  DisableCoverage=on
  GFLIB_ControllerPIpAW_SF : S-Function  FunctionName=GFLIB_ControllerPIpAW_SF_FLT  Parameters=showStates,resetStatesEnable,fltPropGain,fltIntegGain,fltLowerLimit,fltUpperLimit  SFunctionDeploymentMode=off  EnableBusSupport=off
  copyright : Subsystem
      mask Display: text(10,90,'FILE:');text(10,75,'DESRIPTION:');text(10,60,'COPYRIGHT:');text(10,45,'VERSION:');text(10,30,'DATE:')
  copyright2 : Subsystem
      mask Display: text(10,90,'GFLIB_ControllerPIpAW_BAM_FLT.mdl');text(10,75,'Parallel form of a standard PI controller with anti-windup.');text(10,60,'NXP 2020');text(10,45,'1.0');text(10,30,'28-Mar-2020');
  fltInK_1 : Ground
  fltInK_1_Out : Terminator
  fltIntegGain : Ground
  fltIntegPartK_1 : Ground
  fltIntegPartK_1_Out : Terminator
  fltLowerLimit : Ground
  fltPropGain : Ground
  fltUpperLimit : Ground
  fltOut : Outport
  u16LimitFlag : Outport  Port=2
  wires:
  GFLIB_ControllerPIpAW_SF/4 -> fltInK_1_Out/1
  GFLIB_ControllerPIpAW_SF/3 -> fltIntegPartK_1_Out/1
  GFLIB_ControllerPIpAW_SF/2 -> u16LimitFlag/1
  GFLIB_ControllerPIpAW_SF/1 -> fltOut/1
  fltInK_1/1 -> GFLIB_ControllerPIpAW_SF/8
  fltIntegPartK_1/1 -> GFLIB_ControllerPIpAW_SF/7
  fltUpperLimit/1 -> GFLIB_ControllerPIpAW_SF/6
  fltLowerLimit/1 -> GFLIB_ControllerPIpAW_SF/5
  fltIntegGain/1 -> GFLIB_ControllerPIpAW_SF/4
  fltPropGain/1 -> GFLIB_ControllerPIpAW_SF/3
  fltControllerPIpAWOut_preset/1 -> GFLIB_ControllerPIpAW_SF/2
  fltInErr/1 -> GFLIB_ControllerPIpAW_SF/1

== system ammclib_bam/GFLIB/FLT/GFLIB_ControllerPIp_FLT ==
  fltInErr : Inport  OutDataTypeStr=single
  fltControllerPIpOut_preset : Inport  Port=2  OutDataTypeStr=single
  Reset : ResetPort  DisableCoverage=on
  GFLIB_ControllerPIp_SF : S-Function  FunctionName=GFLIB_ControllerPIp_SF_FLT  Parameters=showStates,resetStatesEnable,fltPropGain,fltIntegGain  SFunctionDeploymentMode=off  EnableBusSupport=off
  copyright : Subsystem
      mask Display: text(10,90,'FILE:');text(10,75,'DESRIPTION:');text(10,60,'COPYRIGHT:');text(10,45,'VERSION:');text(10,30,'DATE:')
  copyright2 : Subsystem
      mask Display: text(10,90,'GFLIB_ControllerPIp_BAM_FLT.mdl');text(10,75,'Parallel form of a standard PI controller without anti-windup.');text(10,60,'NXP 2020');text(10,45,'1.0');text(10,30,'28-Mar-2020');
  fltInK_1 : Ground
  fltInK_1_Out : Terminator
  fltIntegGain : Ground
  fltIntegPartK_1 : Ground
  fltIntegPartK_1_Out : Terminator
  fltPropGain : Ground
  fltOut : Outport
  wires:
  GFLIB_ControllerPIp_SF/3 -> fltInK_1_Out/1
  GFLIB_ControllerPIp_SF/2 -> fltIntegPartK_1_Out/1
  GFLIB_ControllerPIp_SF/1 -> fltOut/1
  fltInK_1/1 -> GFLIB_ControllerPIp_SF/6
  fltIntegPartK_1/1 -> GFLIB_ControllerPIp_SF/5
  fltIntegGain/1 -> GFLIB_ControllerPIp_SF/4
  fltPropGain/1 -> GFLIB_ControllerPIp_SF/3
  fltControllerPIpOut_preset/1 -> GFLIB_ControllerPIp_SF/2
  fltInErr/1 -> GFLIB_ControllerPIp_SF/1

== system ammclib_bam/GFLIB/FLT/GFLIB_ControllerPIrAW_FLT ==
  fltInErr : Inport  OutDataTypeStr=single
  fltControllerPIrAWOut_preset : Inport  Port=2  OutDataTypeStr=single
  Reset : ResetPort  DisableCoverage=on
  GFLIB_ControllerPIrAW_SF : S-Function  FunctionName=GFLIB_ControllerPIrAW_SF_FLT  Parameters=showStates,resetStatesEnable,fltUpperLimit,fltLowerLimit,fltCC1sc,fltCC2sc  SFunctionDeploymentMode=off  EnableBusSupport=off
  copyright : Subsystem
      mask Display: text(10,90,'FILE:');text(10,75,'DESRIPTION:');text(10,60,'COPYRIGHT:');text(10,45,'VERSION:');text(10,30,'DATE:')
  copyright2 : Subsystem
      mask Display: text(10,90,'GFLIB_ControllerPIrAW_BAM_FLT.mdl');text(10,75,'Recurrent form PI controller with anti-windup.');text(10,60,'NXP 2020');text(10,45,'1.0');text(10,30,'28-Mar-2020');
  fltAcc : Ground
  fltAcc_Out : Terminator
  fltCC1sc : Ground
  fltCC2sc : Ground
  fltInErrK1 : Ground
  fltInErrK1_Out : Terminator
  fltLowerLimit : Ground
  fltUpperLimit : Ground
  fltOut : Outport
  wires:
  GFLIB_ControllerPIrAW_SF/3 -> fltInErrK1_Out/1
  GFLIB_ControllerPIrAW_SF/2 -> fltAcc_Out/1
  GFLIB_ControllerPIrAW_SF/1 -> fltOut/1
  fltCC2sc/1 -> GFLIB_ControllerPIrAW_SF/8
  fltCC1sc/1 -> GFLIB_ControllerPIrAW_SF/7
  fltInErrK1/1 -> GFLIB_ControllerPIrAW_SF/6
  fltAcc/1 -> GFLIB_ControllerPIrAW_SF/5
  fltLowerLimit/1 -> GFLIB_ControllerPIrAW_SF/4
  fltUpperLimit/1 -> GFLIB_ControllerPIrAW_SF/3
  fltControllerPIrAWOut_preset/1 -> GFLIB_ControllerPIrAW_SF/2
  fltInErr/1 -> GFLIB_ControllerPIrAW_SF/1

== system ammclib_bam/GFLIB/FLT/GFLIB_ControllerPIr_FLT ==
  fltInErr : Inport  OutDataTypeStr=single
  fltControllerPIrOut_preset : Inport  Port=2  OutDataTypeStr=single
  Reset : ResetPort  DisableCoverage=on
  GFLIB_ControllerPIr_SF : S-Function  FunctionName=GFLIB_ControllerPIr_SF_FLT  Parameters=showStates,resetStatesEnable,fltCC1,fltCC2  SFunctionDeploymentMode=off  EnableBusSupport=off
  copyright : Subsystem
      mask Display: text(10,90,'FILE:');text(10,75,'DESRIPTION:');text(10,60,'COPYRIGHT:');text(10,45,'VERSION:');text(10,30,'DATE:')
  copyright2 : Subsystem
      mask Display: text(10,90,'GFLIB_ControllerPIr_BAM_FLT.mdl');text(10,75,'Recurrent form PI controller without anti-windup.');text(10,60,'NXP 2020');text(10,45,'1.0');text(10,30,'28-Mar-2020');
  fltAcc : Ground
  fltAcc_Out : Terminator
  fltCC1sc : Ground
  fltCC2sc : Ground
  fltInErrK1 : Ground
  fltInErrK1_Out : Terminator
  fltOut : Outport
  wires:
  GFLIB_ControllerPIr_SF/3 -> fltInErrK1_Out/1
  GFLIB_ControllerPIr_SF/2 -> fltAcc_Out/1
  GFLIB_ControllerPIr_SF/1 -> fltOut/1
  fltInErrK1/1 -> GFLIB_ControllerPIr_SF/6
  fltAcc/1 -> GFLIB_ControllerPIr_SF/5
  fltCC2sc/1 -> GFLIB_ControllerPIr_SF/4
  fltCC1sc/1 -> GFLIB_ControllerPIr_SF/3
  fltControllerPIrOut_preset/1 -> GFLIB_ControllerPIr_SF/2
  fltInErr/1 -> GFLIB_ControllerPIr_SF/1

== system ammclib_bam/GFLIB/FLT/GFLIB_Cos_FLT ==
  fltIn : Inport  OutDataTypeStr=single
  GFLIB_Cos_SF : S-Function  FunctionName=GFLIB_Cos_SF_FLT  SFunctionDeploymentMode=off  EnableBusSupport=off
  copyright : Subsystem
      mask Display: text(10,90,'FILE:');text(10,75,'DESRIPTION:');text(10,60,'COPYRIGHT:');text(10,45,'VERSION:');text(10,30,'DATE:')
  copyright2 : Subsystem
      mask Display: text(10,90,'GFLIB_Cos_BAM_FLT.mdl');text(10,75,'Cosine function');text(10,60,'NXP 2020');text(10,45,'1.0');text(10,30,'18-Mar-2020');
  fltOut : Outport
  wires:
  GFLIB_Cos_SF/1 -> fltOut/1
  fltIn/1 -> GFLIB_Cos_SF/1

== system ammclib_bam/GFLIB/FLT/GFLIB_Hyst_FLT ==
  fltIn : Inport  OutDataTypeStr=single
  GFLIB_Hyst_SF : S-Function  FunctionName=GFLIB_Hyst_SF_FLT  Parameters=showStates,fltHystOn,fltHystOff,fltOutValOn,fltOutValOff  SFunctionDeploymentMode=off  EnableBusSupport=off
  copyright : Subsystem
      mask Display: text(10,90,'FILE:');text(10,75,'DESRIPTION:');text(10,60,'COPYRIGHT:');text(10,45,'VERSION:');text(10,30,'DATE:')
  copyright2 : Subsystem
      mask Display: text(10,90,'GFLIB_Hyst_BAM_FLT.mdl');text(10,75,'Hysteresis function.');text(10,60,'NXP 2020');text(10,45,'1.0');text(10,30,'18-Mar-2020');
  fltHystOff : Ground
  fltHystOn : Ground
  fltOutState : Ground
  fltOutState_Out : Terminator
  fltOutValOff : Ground
  fltOutValOn : Ground
  fltOut : Outport
  wires:
  GFLIB_Hyst_SF/2 -> fltOutState_Out/1
  GFLIB_Hyst_SF/1 -> fltOut/1
  fltOutState/1 -> GFLIB_Hyst_SF/6
  fltOutValOff/1 -> GFLIB_Hyst_SF/5
  fltOutValOn/1 -> GFLIB_Hyst_SF/4
  fltHystOff/1 -> GFLIB_Hyst_SF/3
  fltHystOn/1 -> GFLIB_Hyst_SF/2
  fltIn/1 -> GFLIB_Hyst_SF/1

== system ammclib_bam/GFLIB/FLT/GFLIB_IntegratorTR_FLT ==
  fltIn : Inport  OutDataTypeStr=single
  fltIntegratorTROut_preset : Inport  Port=2  OutDataTypeStr=single
  Reset : ResetPort  DisableCoverage=on
  GFLIB_IntegratorTR_SF : S-Function  FunctionName=GFLIB_IntegratorTR_SF_FLT  Parameters=showStates,resetStatesEnable,fltC1  SFunctionDeploymentMode=off  EnableBusSupport=off
  copyright : Subsystem
      mask Display: text(10,90,'FILE:');text(10,75,'DESRIPTION:');text(10,60,'COPYRIGHT:');text(10,45,'VERSION:');text(10,30,'DATE:')
  copyright2 : Subsystem
      mask Display: text(10,90,'GFLIB_IntegratorTR_BAM_FLT.mdl');text(10,75,'Discrete integrator transformed from a linear model using Billinear (trapezoidal) transformation.');text(10,60,'NXP 2020');text(10,45,'1.0');text(10,30,'28-Mar-2020');
  fltC1 : Ground
  fltInK1 : Ground
  fltInK1_Out : Terminator
  fltState : Ground
  fltState_Out : Terminator
  fltOut : Outport
  wires:
  GFLIB_IntegratorTR_SF/3 -> fltInK1_Out/1
  GFLIB_IntegratorTR_SF/2 -> fltState_Out/1
  GFLIB_IntegratorTR_SF/1 -> fltOut/1
  fltInK1/1 -> GFLIB_IntegratorTR_SF/5
  fltState/1 -> GFLIB_IntegratorTR_SF/4
  fltC1/1 -> GFLIB_IntegratorTR_SF/3
  fltIntegratorTROut_preset/1 -> GFLIB_IntegratorTR_SF/2
  fltIn/1 -> GFLIB_IntegratorTR_SF/1

== system ammclib_bam/GFLIB/FLT/GFLIB_Limit_FLT ==
  fltIn : Inport  OutDataTypeStr=single
  GFLIB_Limit_SF : S-Function  FunctionName=GFLIB_Limit_SF_FLT  Parameters=showStates,fltLowerLimit,fltUpperLimit  SFunctionDeploymentMode=off  EnableBusSupport=off
  copyright : Subsystem
      mask Display: text(10,90,'FILE:');text(10,75,'DESRIPTION:');text(10,60,'COPYRIGHT:');text(10,45,'VERSION:');text(10,30,'DATE:')
  copyright2 : Subsystem
      mask Display: text(10,90,'GFLIB_Limit_BAM_FLT.mdl');text(10,75,'Limit function.');text(10,60,'NXP 2020');text(10,45,'1.0');text(10,30,'23-Mar-2020');
  fltLowerLimit : Ground
  fltUpperLimit : Ground
  fltOut : Outport
  wires:
  GFLIB_Limit_SF/1 -> fltOut/1
  fltUpperLimit/1 -> GFLIB_Limit_SF/3
  fltLowerLimit/1 -> GFLIB_Limit_SF/2
  fltIn/1 -> GFLIB_Limit_SF/1

== system ammclib_bam/GFLIB/FLT/GFLIB_Log10_FLT ==
  fltIn : Inport  OutDataTypeStr=single
  GFLIB_Log10_SF : S-Function  FunctionName=GFLIB_Log10_SF_FLT  SFunctionDeploymentMode=off  EnableBusSupport=off
  copyright : Subsystem
      mask Display: text(10,90,'FILE:');text(10,75,'DESRIPTION:');text(10,60,'COPYRIGHT:');text(10,45,'VERSION:');text(10,30,'DATE:')
  copyright2 : Subsystem
      mask Display: text(10,90,'GFLIB_Log10_BAM_FLT.mdl');text(10,75,'Fast base-10 logarithm');text(10,60,'NXP 2020');text(10,45,'1.0');text(10,30,'18-Mar-2020');
  fltOut : Outport
  wires:
  GFLIB_Log10_SF/1 -> fltOut/1
  fltIn/1 -> GFLIB_Log10_SF/1

== system ammclib_bam/GFLIB/FLT/GFLIB_LowerLimit_FLT ==
  fltIn : Inport  OutDataTypeStr=single
  GFLIB_LowerLimit_SF : S-Function  FunctionName=GFLIB_LowerLimit_SF_FLT  Parameters=showStates,fltLowerLimit  SFunctionDeploymentMode=off  EnableBusSupport=off
  copyright : Subsystem
      mask Display: text(10,90,'FILE:');text(10,75,'DESRIPTION:');text(10,60,'COPYRIGHT:');text(10,45,'VERSION:');text(10,30,'DATE:')
  copyright2 : Subsystem
      mask Display: text(10,90,'GFLIB_LowerLimit_BAM_FLT.mdl');text(10,75,'Lower limit function.');text(10,60,'NXP 2020');text(10,45,'1.0');text(10,30,'18-Mar-2020');
  fltLowerLimit : Ground
  fltOut : Outport
  wires:
  GFLIB_LowerLimit_SF/1 -> fltOut/1
  fltLowerLimit/1 -> GFLIB_LowerLimit_SF/2
  fltIn/1 -> GFLIB_LowerLimit_SF/1

== system ammclib_bam/GFLIB/FLT/GFLIB_Lut1D_FLT ==
  fltIn : Inport  OutDataTypeStr=single
  u32ShamOffset : Inport  Port=2  OutDataTypeStr=uint32
  GFLIB_Lut1D_SF : S-Function  FunctionName=GFLIB_Lut1D_SF_FLT  Parameters=pfltTable,s32MidIdx  SFunctionDeploymentMode=off  EnableBusSupport=off
  copyright : Subsystem
      mask Display: text(10,90,'FILE:');text(10,75,'DESRIPTION:');text(10,60,'COPYRIGHT:');text(10,45,'VERSION:');text(10,30,'DATE:')
  copyright2 : Subsystem
      mask Display: text(10,90,'GFLIB_Lut1D_BAM_FLT.mdl');text(10,75,'One dimensional lookup table function');text(10,60,'NXP 2020');text(10,45,'1.0');text(10,30,'23-Mar-2020');
  fltOut : Outport
  wires:
  GFLIB_Lut1D_SF/1 -> fltOut/1
  u32ShamOffset/1 -> GFLIB_Lut1D_SF/2
  fltIn/1 -> GFLIB_Lut1D_SF/1

== system ammclib_bam/GFLIB/FLT/GFLIB_Lut2D_FLT ==
  fltIn1 : Inport  OutDataTypeStr=single
  fltIn2 : Inport  Port=2  OutDataTypeStr=single
  u32ShamOffset1 : Inport  Port=3  OutDataTypeStr=uint32
  u32ShamOffset2 : Inport  Port=4  OutDataTypeStr=uint32
  GFLIB_Lut2D_SF : S-Function  FunctionName=GFLIB_Lut2D_SF_FLT  Parameters=pfltTable,s32MidIdx  SFunctionDeploymentMode=off  EnableBusSupport=off
  copyright : Subsystem
      mask Display: text(10,90,'FILE:');text(10,75,'DESRIPTION:');text(10,60,'COPYRIGHT:');text(10,45,'VERSION:');text(10,30,'DATE:')
  copyright2 : Subsystem
      mask Display: text(10,90,'GFLIB_Lut2D_BAM_FLT.mdl');text(10,75,'Two dimensional lookup table function');text(10,60,'NXP 2020');text(10,45,'1.0');text(10,30,'23-Mar-2020');
  fltOut : Outport
  wires:
  GFLIB_Lut2D_SF/1 -> fltOut/1
  u32ShamOffset2/1 -> GFLIB_Lut2D_SF/4
  u32ShamOffset1/1 -> GFLIB_Lut2D_SF/3
  fltIn2/1 -> GFLIB_Lut2D_SF/2
  fltIn1/1 -> GFLIB_Lut2D_SF/1

== system ammclib_bam/GFLIB/FLT/GFLIB_Ramp_FLT ==
  fltIn : Inport  OutDataTypeStr=single
  GFLIB_Ramp_SF : S-Function  FunctionName=GFLIB_Ramp_SF_FLT  Parameters=showStates,fltRampUp,fltRampDown  SFunctionDeploymentMode=off  EnableBusSupport=off
  copyright : Subsystem
      mask Display: text(10,90,'FILE:');text(10,75,'DESRIPTION:');text(10,60,'COPYRIGHT:');text(10,45,'VERSION:');text(10,30,'DATE:')
  copyright2 : Subsystem
      mask Display: text(10,90,'GFLIB_Ramp_BAM_FLT.mdl');text(10,75,'Rate of change limiter - ramp function.');text(10,60,'NXP 2020');text(10,45,'1.0');text(10,30,'18-Mar-2020');
  fltRampDown : Ground
  fltRampUp : Ground
  fltState : Ground
  fltState_Out : Terminator
  fltOut : Outport
  wires:
  GFLIB_Ramp_SF/2 -> fltState_Out/1
  GFLIB_Ramp_SF/1 -> fltOut/1
  fltRampDown/1 -> GFLIB_Ramp_SF/4
  fltRampUp/1 -> GFLIB_Ramp_SF/3
  fltState/1 -> GFLIB_Ramp_SF/2
  fltIn/1 -> GFLIB_Ramp_SF/1

== system ammclib_bam/GFLIB/FLT/GFLIB_Sign_FLT ==
  fltIn : Inport  OutDataTypeStr=single
  GFLIB_Sign_SF : S-Function  FunctionName=GFLIB_Sign_SF_FLT  SFunctionDeploymentMode=off  EnableBusSupport=off
  copyright : Subsystem
      mask Display: text(10,90,'FILE:');text(10,75,'DESRIPTION:');text(10,60,'COPYRIGHT:');text(10,45,'VERSION:');text(10,30,'DATE:')
  copyright2 : Subsystem
      mask Display: text(10,90,'GFLIB_Sign_BAM_FLT.mdl');text(10,75,'Sign function.');text(10,60,'NXP 2020');text(10,45,'1.0');text(10,30,'18-Mar-2020');
  fltOut : Outport
  wires:
  GFLIB_Sign_SF/1 -> fltOut/1
  fltIn/1 -> GFLIB_Sign_SF/1

== system ammclib_bam/GFLIB/FLT/GFLIB_SinCos_FLT ==
  fltIn : Inport  OutDataTypeStr=single
  GFLIB_SinCos_SF : S-Function  FunctionName=GFLIB_SinCos_SF_FLT  SFunctionDeploymentMode=off  EnableBusSupport=off
  copyright : Subsystem
      mask Display: text(10,90,'FILE:');text(10,75,'DESRIPTION:');text(10,60,'COPYRIGHT:');text(10,45,'VERSION:');text(10,30,'DATE:')
  copyright2 : Subsystem
      mask Display: text(10,90,'GFLIB_SinCos_BAM_FLT.mdl');text(10,75,'Sine and cosine of the same argument');text(10,60,'NXP 2020');text(10,45,'1.0');text(10,30,'18-Mar-2020');
  pOut : Outport
  wires:
  GFLIB_SinCos_SF/1 -> pOut/1
  fltIn/1 -> GFLIB_SinCos_SF/1

== system ammclib_bam/GFLIB/FLT/GFLIB_Sin_FLT ==
  fltIn : Inport  OutDataTypeStr=single
  GFLIB_Sin_SF : S-Function  FunctionName=GFLIB_Sin_SF_FLT  SFunctionDeploymentMode=off  EnableBusSupport=off
  copyright : Subsystem
      mask Display: text(10,90,'FILE:');text(10,75,'DESRIPTION:');text(10,60,'COPYRIGHT:');text(10,45,'VERSION:');text(10,30,'DATE:')
  copyright2 : Subsystem
      mask Display: text(10,90,'GFLIB_Sin_BAM_FLT.mdl');text(10,75,'Sine function');text(10,60,'NXP 2020');text(10,45,'1.0');text(10,30,'18-Mar-2020');
  fltOut : Outport
  wires:
  GFLIB_Sin_SF/1 -> fltOut/1
  fltIn/1 -> GFLIB_Sin_SF/1

== system ammclib_bam/GFLIB/FLT/GFLIB_Sqrt_FLT ==
  fltIn : Inport  OutDataTypeStr=single
  GFLIB_Sqrt_SF : S-Function  FunctionName=GFLIB_Sqrt_SF_FLT  SFunctionDeploymentMode=off  EnableBusSupport=off
  copyright : Subsystem
      mask Display: text(10,90,'FILE:');text(10,75,'DESRIPTION:');text(10,60,'COPYRIGHT:');text(10,45,'VERSION:');text(10,30,'DATE:')
  copyright2 : Subsystem
      mask Display: text(10,90,'GFLIB_Sqrt_BAM_FLT.mdl');text(10,75,'Square root approximation.');text(10,60,'NXP 2020');text(10,45,'1.0');text(10,30,'18-Mar-2020');
  fltOut : Outport
  wires:
  GFLIB_Sqrt_SF/1 -> fltOut/1
  fltIn/1 -> GFLIB_Sqrt_SF/1

== system ammclib_bam/GFLIB/FLT/GFLIB_Tan_FLT ==
  fltIn : Inport  OutDataTypeStr=single
  GFLIB_Tan_SF : S-Function  FunctionName=GFLIB_Tan_SF_FLT  SFunctionDeploymentMode=off  EnableBusSupport=off
  copyright : Subsystem
      mask Display: text(10,90,'FILE:');text(10,75,'DESRIPTION:');text(10,60,'COPYRIGHT:');text(10,45,'VERSION:');text(10,30,'DATE:')
  copyright2 : Subsystem
      mask Display: text(10,90,'GFLIB_Tan_BAM_FLT.mdl');text(10,75,'Trigonometric tangent function');text(10,60,'NXP 2020');text(10,45,'1.0');text(10,30,'18-Mar-2020');
  fltOut : Outport
  wires:
  GFLIB_Tan_SF/1 -> fltOut/1
  fltIn/1 -> GFLIB_Tan_SF/1

== system ammclib_bam/GFLIB/FLT/GFLIB_UpperLimit_FLT ==
  fltIn : Inport  OutDataTypeStr=single
  GFLIB_UpperLimit_SF : S-Function  FunctionName=GFLIB_UpperLimit_SF_FLT  Parameters=showStates,fltUpperLimit  SFunctionDeploymentMode=off  EnableBusSupport=off
  copyright : Subsystem
      mask Display: text(10,90,'FILE:');text(10,75,'DESRIPTION:');text(10,60,'COPYRIGHT:');text(10,45,'VERSION:');text(10,30,'DATE:')
  copyright2 : Subsystem
      mask Display: text(10,90,'GFLIB_UpperLimit_BAM_FLT.mdl');text(10,75,'Upper limit function.');text(10,60,'NXP 2020');text(10,45,'1.0');text(10,30,'23-Mar-2020');
  fltUpperLimit : Ground
  fltOut : Outport
  wires:
  GFLIB_UpperLimit_SF/1 -> fltOut/1
  fltUpperLimit/1 -> GFLIB_UpperLimit_SF/2
  fltIn/1 -> GFLIB_UpperLimit_SF/1

== system ammclib_bam/GFLIB/FLT/GFLIB_VLog10_FLT ==
  pIn : Inport  OutDataTypeStr=single
  GFLIB_VLog10_SF : S-Function  FunctionName=GFLIB_VLog10_SF_FLT  SFunctionDeploymentMode=off  EnableBusSupport=off
  copyright : Subsystem
      mask Display: text(10,90,'FILE:');text(10,75,'DESRIPTION:');text(10,60,'COPYRIGHT:');text(10,45,'VERSION:');text(10,30,'DATE:')
  copyright2 : Subsystem
      mask Display: text(10,90,'GFLIB_VLog10_BAM_FLT.mdl');text(10,75,'Vector base-10 logarithm');text(10,60,'NXP 2020');text(10,45,'1.0');text(10,30,'18-Mar-2020');
  pOut : Outport
  wires:
  GFLIB_VLog10_SF/1 -> pOut/1
  pIn/1 -> GFLIB_VLog10_SF/1
